simulink library "INT_Tra_RtnIntfc"  (R2016b)
settings: Solver=VariableStepAuto  StartTime=0.0  StopTime=10.0  RelTol=1e-3
settings Model: Creator=Administrator  LastModifiedBy=Administrator

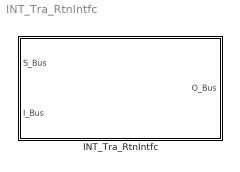
== system INT_Tra_RtnIntfc ==
  INT_Tra_RtnIntfc : Subsystem

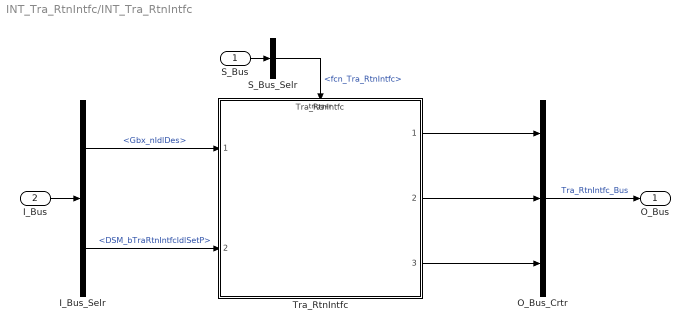
== system INT_Tra_RtnIntfc/INT_Tra_RtnIntfc ==
  S_Bus : Inport
  I_Bus : Inport  Port=2
  I_Bus_Selr : BusSelector  OutputSignals=Gbx_nIdlDes,DSM_bTraRtnIntfcIdlSetP
  O_Bus_Crtr : BusCreator  Inputs=3
  S_Bus_Selr : BusSelector  OutputSignals=fcn_Tra_RtnIntfc
  Tra_RtnIntfc : ModelReference  ModelNameDialog=Tra_RtnIntfc  SimulationMode=Normal  ModelReferenceVersion=1.13  TriggerPortName=function  TriggerPortTriggerType=function-call  TriggerPortStatesWhenEnabling=held
  O_Bus : Outport
  wires:
  S_Bus_Selr/1 -> Tra_RtnIntfc/Trigger  "<fcn_Tra_RtnIntfc>"
  S_Bus/1 -> S_Bus_Selr/1
  I_Bus/1 -> I_Bus_Selr/1
  I_Bus_Selr/1 -> Tra_RtnIntfc/1  "<Gbx_nIdlDes>"
  I_Bus_Selr/2 -> Tra_RtnIntfc/2  "<DSM_bTraRtnIntfcIdlSetP>"
  O_Bus_Crtr/1 -> O_Bus/1  "Tra_RtnIntfc_Bus"
  Tra_RtnIntfc/1 -> O_Bus_Crtr/1
  Tra_RtnIntfc/2 -> O_Bus_Crtr/2
  Tra_RtnIntfc/3 -> O_Bus_Crtr/3
